simulink model "gm_sampleModel1849_sub"  (R2023a)
settings: Solver=VariableStepAuto  StartTime=0.0  StopTime=10.0  RelTol=1e-3
libraries: simulink x2
settings Model: Creator=user1  LastModifiedBy=user1
settings OptimizationCC: BlockReduction=off  ConditionallyExecuteInputs=off
settings DebuggingCC: InheritedTsInSrcMsg=none

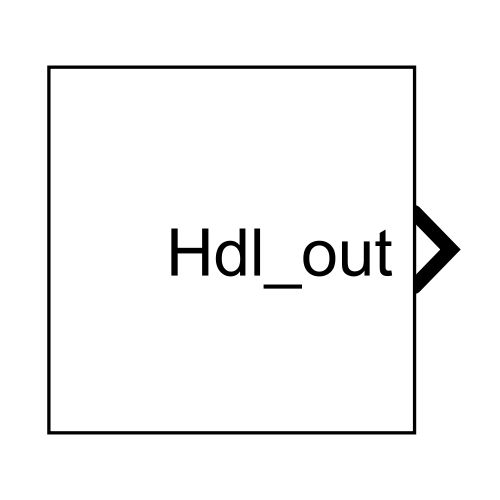
[thumbnail: Simulink's stored preview of the top-level diagram]
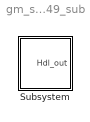
== system gm_sampleModel1849_sub ==
  Subsystem : Subsystem

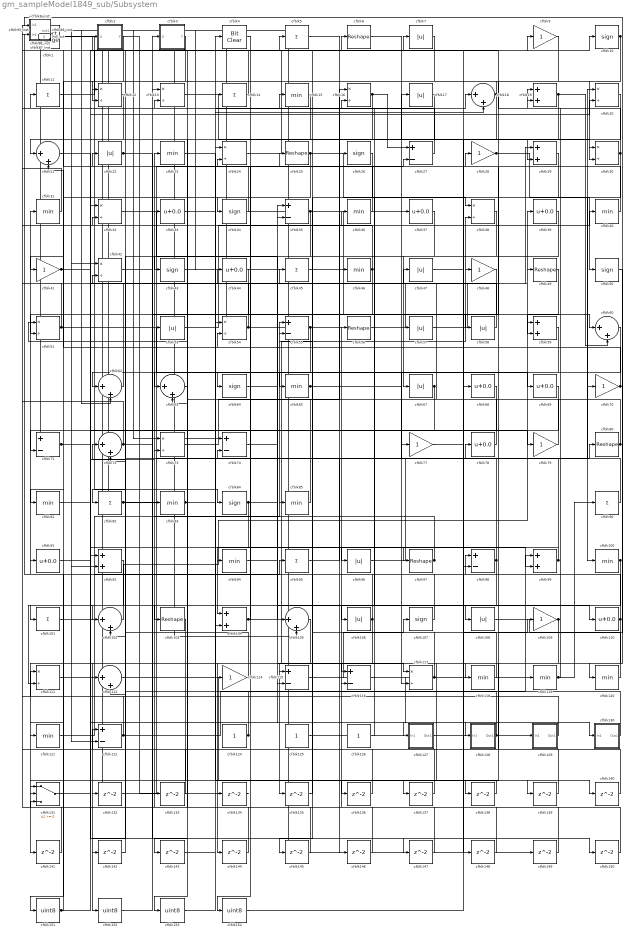
== system gm_sampleModel1849_sub/Subsystem ==
  cfblk1 : simulink/Logic and Bit Operations/Detect Change  vinit=0  OutDataTypeStr=uint8
      settings: LibrarySourceBlock=|
      | hdlsllib/Logic and Bit
      | Operations/Detect
      | Change
  cfblk{10,26,34,43,50,64,84,107} (8 alike) : Signum
  cfblk{15,23,31,36,40,46,65,81,83,85,94,100,118..121} (16 alike) : MinMax  OutDataTypeStr=uint8
  cfblk{5,11,14,45,82,90,95,101} (8 alike) : Sum  Inputs=+  OutDataTypeStr=uint8
  cfblk{18,21,60,62..63,72,102,105,112} (9 alike) : Sum  Inputs=|++  OutDataTypeStr=uint8
  cfblk{6,25,49,56,80,97,103} (7 alike) : Reshape
  cfblk{19,29,59,92,99,104} (6 alike) : Sum  OutDataTypeStr=uint8
  cfblk{7,17,22,47,53,57..58,67,96,106,108} (11 alike) : Abs  OutDataTypeStr=uint8  SaturateOnIntegerOverflow=off
  cfblk{9,28,41,48,70,77,79,109,114} (9 alike) : Gain  OutDataTypeStr=uint8
  cfblk{33,37,39,44,68..69,78,91,110} (9 alike) : Bias  Bias=0.0  SaturateOnIntegerOverflow=off
  cfblk{12..13,16,20,24,30,32,38,42,51,54,73,111,117} (14 alike) : Product  Inputs=*/  OutDataTypeStr=uint8  RndMeth=Zero  SaturateOnIntegerOverflow=on
  cfblk113_inst : Subsystem
  cfblk{27,35,55,71,74,98,115..116,122} (9 alike) : Sum  Inputs=+-  OutDataTypeStr=uint8
  cfblk124 : Constant  OutDataTypeStr=uint8  SampleTime=-1
  cfblk125 : Constant  OutDataTypeStr=uint8  SampleTime=-1
  cfblk126 : Constant  OutDataTypeStr=uint8  SampleTime=-1
  cfblk127 : Subsystem
  cfblk128 : Subsystem
  cfblk129 : Subsystem
  cfblk130 : Subsystem
  cfblk131 : Switch  OutDataTypeStr=uint8  SaturateOnIntegerOverflow=off  InputSameDT=off
  cfblk{132..150} (19 alike) : Delay  SampleTime=1
  cfblk{151..154} (4 alike) : DataTypeConversion  OutDataTypeStr=uint8  SaturateOnIntegerOverflow=off  RndMeth=Floor
  cfblk2 : Subsystem  mask(Detect Fall Nonpositive){vinit=double(0), InputProcessing=Elements as channels (sample based), OutDataTypeStr=uint8}
      mask prompts: vinit "Simulink:masks:InitialCondition_MP"; InputProcessing "Simulink:masks:InputProcessing_MP"; OutDataTypeStr "Simulink:masks:OutputDataType_MP"
      mask help: Simulink:masks:DetectFallNonpositive_MD
      mask init:
      | InputProcessing = 'Elements as channels (sample based)';
      | OutDataTypeStr = 'uint8';
      | vinit = double(0);
      mask TypeOptions InputProcessing: Simulink:masks:ColumnsAsChannelsFrameBased | Simulink:masks:ElementsAsChannelsSampleBased
      mask TypeOptions OutDataTypeStr: Simulink:masks:uint8 | Simulink:masks:boolean
      mask Display: fprintf('U <= 0\n&  NOT\nU/z <= 0')
  cfblk3 : Subsystem  mask(Detect Rise Positive){vinit=double(0), InputProcessing=Elements as channels (sample based), OutDataTypeStr=uint8}
      mask prompts: vinit "Simulink:masks:InitialCondition_MP"; InputProcessing "Simulink:masks:InputProcessing_MP"; OutDataTypeStr "Simulink:masks:OutputDataType_MP"
      mask help: Simulink:masks:DetectRisePositive_MD
      mask init:
      | InputProcessing = 'Elements as channels (sample based)';
      | OutDataTypeStr = 'uint8';
      | vinit = double(0);
      mask TypeOptions InputProcessing: Simulink:masks:ColumnsAsChannelsFrameBased | Simulink:masks:ElementsAsChannelsSampleBased
      mask TypeOptions OutDataTypeStr: Simulink:masks:uint8 | Simulink:masks:boolean
      mask Display: fprintf('U > 0\n&  NOT\nU/z > 0')
  cfblk4 : simulink/Logic and Bit Operations/Bit Clear  iBit=0
      settings: LibrarySourceBlock=|
      | hdlsllib/Logic and Bit
      | Operations/Bit Clear
  cfblk52_inst : Subsystem
  cfblk61_inst : Subsystem
  cfblk66_inst : Subsystem
  cfblk75_inst : Subsystem
  cfblk76_inst : Subsystem
  cfblk86_inst : Subsystem
  cfblk87_inst : Subsystem
  cfblk88_inst : Subsystem
  cfblk89_inst : Subsystem
  cfblk8_inst : Subsystem
  cfblk93_inst : Subsystem
  Hdl_out : Outport  OutDataTypeStr=uint8  SampleTime=1
  wires:
  cfblk1/1 -> cfblk84/1
  cfblk10/1 -> cfblk30/2, cfblk12/2
  cfblk100/1 -> cfblk112/2, cfblk108/1
  cfblk101/1 -> cfblk55/1
  cfblk102/1 -> cfblk39/1
  cfblk103/1 -> cfblk152/1
  cfblk104/1 -> cfblk35/2, cfblk38/2, cfblk24/2, cfblk117/1
  cfblk105/1 -> cfblk144/1
  cfblk106/1 -> cfblk141/1, cfblk31/1
  cfblk107/1 -> cfblk89_inst/2(in2)
  cfblk108/1 -> cfblk89_inst/1(in1)
  cfblk109/1 -> cfblk19/1, cfblk118/1
  cfblk11/1 -> cfblk6/1
  cfblk110/1 -> cfblk138/1, cfblk137/1, cfblk135/1, cfblk23/1, cfblk45/1
  cfblk111/1 -> cfblk132/1
  cfblk112/1 -> cfblk139/1
  cfblk113_inst/1(out1) -> cfblk129/1(In1)
  cfblk114/1 -> cfblk11/1
  cfblk115/1 -> cfblk107/1
  cfblk116/1 -> cfblk128/1(In1)
  cfblk117/1 -> cfblk74/2, cfblk109/1
  cfblk118/1 -> cfblk85/1
  cfblk119/1 -> cfblk19/2, cfblk90/1
  cfblk12/1 -> cfblk51/2
  cfblk120/1 -> cfblk78/1
  cfblk121/1 -> cfblk95/1
  cfblk122/1 -> cfblk99/1, cfblk88_inst/2(in2), cfblk8_inst/1(in1)
  cfblk124/1 -> cfblk32/2, cfblk13/2
  cfblk125/1 -> cfblk56/1
  cfblk126/1 -> cfblk16/2
  cfblk127/1(Out1) -> cfblk10/1
  cfblk128/1(Out1) -> cfblk22/1, cfblk5/1
  cfblk129/1(Out1) -> cfblk111/1
  cfblk13/1 -> cfblk146/1
  cfblk130/1(Out1) -> cfblk28/1
  cfblk131/1 -> cfblk48/1
  cfblk132/1 -> cfblk27/2
  cfblk133/1 -> cfblk122/1
  cfblk134/1 -> cfblk1/1
  cfblk135/1 -> cfblk55/2
  cfblk136/1 -> cfblk75_inst/2(in2)
  cfblk137/1 -> cfblk72/1
  cfblk138/1 -> cfblk131/2
  cfblk139/1 -> cfblk98/1
  cfblk14/1 -> cfblk88_inst/1(in1)
  cfblk140/1 -> cfblk93_inst/1(in1)
  cfblk141/1 -> cfblk52_inst/1(in1)
  cfblk142/1 -> cfblk102/2
  cfblk143/1 -> cfblk18/2
  cfblk144/1 -> cfblk73/1
  cfblk145/1 -> cfblk66_inst/2(in2)
  cfblk146/1 -> cfblk42/2
  cfblk147/1 -> cfblk63/2
  cfblk148/1 -> cfblk87_inst/1(in1)
  cfblk149/1 -> cfblk131/3
  cfblk15/1 -> cfblk121/1
  cfblk150/1 -> cfblk116/2
  cfblk151/1 -> cfblk91/1, cfblk73/2
  cfblk152/1 -> cfblk3/1(U)
  cfblk153/1 -> cfblk4/1
  cfblk154/1 -> cfblk68/1
  cfblk16/1 -> cfblk43/1, cfblk27/1
  cfblk17/1 -> cfblk34/1
  cfblk18/1 -> cfblk98/2, cfblk12/1
  cfblk19/1 -> cfblk60/2, cfblk143/1
  cfblk2/1(Y) -> cfblk21/1
  cfblk20/1 -> cfblk64/1
  cfblk21/1 -> cfblk96/1
  cfblk22/1 -> cfblk60/1, cfblk150/1
  cfblk23/1 -> cfblk136/1
  cfblk24/1 -> cfblk7/1
  cfblk25/1 -> cfblk41/1, cfblk38/1
  cfblk26/1 -> cfblk65/1
  cfblk27/1 -> cfblk75_inst/1(in1)
  cfblk28/1 -> cfblk50/1, cfblk70/1
  cfblk29/1 -> cfblk106/1
  cfblk3/1(Y) -> cfblk151/1
  cfblk30/1 -> cfblk52_inst/2(in2), cfblk145/1
  cfblk31/1 -> cfblk61_inst/1(in1)
  cfblk32/1 -> cfblk105/1
  cfblk33/1 -> cfblk18/1
  cfblk34/1 -> cfblk86_inst/1(in1)
  cfblk35/1 -> cfblk63/1, cfblk59/2
  cfblk36/1 -> cfblk24/1
  cfblk37/1 -> cfblk153/1
  cfblk38/1 -> cfblk112/1
  cfblk39/1 -> cfblk67/1
  cfblk4/1 -> cfblk154/1
  cfblk40/1 -> cfblk16/1
  cfblk41/1 -> cfblk92/1, cfblk127/1(In1)
  cfblk42/1 -> cfblk33/1
  cfblk43/1 -> cfblk14/1
  cfblk44/1 -> cfblk131/1
  cfblk45/1 -> cfblk100/1
  cfblk46/1 -> cfblk86_inst/2(in2), cfblk82/1
  cfblk47/1 -> cfblk140/1
  cfblk48/1 -> cfblk101/1
  cfblk49/1 -> cfblk59/1
  cfblk5/1 -> cfblk29/2
  cfblk50/1 -> cfblk120/1
  cfblk51/1 -> cfblk113_inst/2(in2), cfblk77/1
  cfblk52_inst/1(out1) -> cfblk93_inst/2(in2), cfblk53/1
  cfblk53/1 -> cfblk36/1
  cfblk54/1 -> cfblk8_inst/2(in2), cfblk116/1
  cfblk55/1 -> cfblk72/2, cfblk62/1
  cfblk56/1 -> cfblk49/1
  cfblk57/1 -> cfblk29/1
  cfblk58/1 -> cfblk32/1
  cfblk59/1 -> cfblk134/1
  cfblk6/1 -> cfblk30/1
  cfblk60/1 -> cfblk142/1
  cfblk61_inst/1(out1) -> cfblk133/1
  cfblk62/1 -> cfblk113_inst/1(in1)
  cfblk63/1 -> cfblk103/1
  cfblk64/1 -> cfblk110/1
  cfblk65/1 -> cfblk69/1, cfblk117/2
  cfblk66_inst/1(out1) -> cfblk87_inst/2(in2), cfblk37/1
  cfblk67/1 -> cfblk71/2, cfblk114/1
  cfblk68/1 -> cfblk115/1
  cfblk69/1 -> cfblk102/1
  cfblk7/1 -> cfblk81/1
  cfblk70/1 -> cfblk21/2, cfblk54/2
  cfblk71/1 -> cfblk79/1, cfblk147/1
  cfblk72/1 -> cfblk99/2, cfblk66_inst/1(in1)
  cfblk73/1 -> cfblk26/1
  cfblk74/1 -> cfblk115/2
  cfblk75_inst/1(out1) -> cfblk42/1
  cfblk76_inst/1(out1) -> cfblk57/1
  cfblk77/1 -> cfblk148/1
  cfblk78/1 -> cfblk2/1(U)
  cfblk79/1 -> cfblk13/1
  cfblk8_inst/1(out1) -> cfblk76_inst/1(in1), cfblk62/2, cfblk105/2
  cfblk80/1 -> cfblk76_inst/2(in2), cfblk47/1
  cfblk81/1 -> cfblk9/1
  cfblk82/1 -> cfblk17/1, cfblk54/1
  cfblk83/1 -> cfblk25/1, Hdl_out/1
  cfblk84/1 -> cfblk104/1, cfblk130/1(In1), cfblk40/1
  cfblk85/1 -> cfblk51/1
  cfblk86_inst/1(out1) -> cfblk71/1, cfblk149/1
  cfblk87_inst/1(out1) -> cfblk122/2, cfblk46/1
  cfblk88_inst/1(out1) -> cfblk74/1
  cfblk89_inst/1(out1) -> cfblk92/2
  cfblk9/1 -> cfblk58/1
  cfblk90/1 -> cfblk15/1
  cfblk91/1 -> cfblk20/2
  cfblk92/1 -> cfblk111/2
  cfblk93_inst/1(out1) -> cfblk119/1
  cfblk94/1 -> cfblk35/1
  cfblk95/1 -> cfblk80/1
  cfblk96/1 -> cfblk20/1
  cfblk97/1 -> cfblk83/1, cfblk94/1
  cfblk98/1 -> cfblk44/1, cfblk104/2
  cfblk99/1 -> cfblk97/1, cfblk61_inst/2(in2)

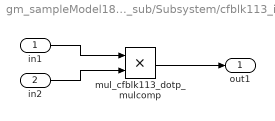
== system gm_sampleModel1849_sub/Subsystem/cfblk113_inst ==
  in1 : Inport  OutDataTypeStr=uint8  SampleTime=1
  in2 : Inport  Port=2  OutDataTypeStr=uint8  SampleTime=1
  mul_cfblk113_dotp_mulcomp : Product  Inputs=**  OutDataTypeStr=uint8  SampleTime=1
  out1 : Outport  OutDataTypeStr=uint8  SampleTime=1
  wires:
  in1/1 -> mul_cfblk113_dotp_mulcomp/1
  in2/1 -> mul_cfblk113_dotp_mulcomp/2
  mul_cfblk113_dotp_mulcomp/1 -> out1/1

== system gm_sampleModel1849_sub/Subsystem/cfblk127 ==
  In1 : Inport  OutDataTypeStr=uint8  PortDimensions=1  SampleTime=1
  Out1 : Outport  SampleTime=1
  wires:
  In1/1 -> Out1/1

== system gm_sampleModel1849_sub/Subsystem/cfblk128 ==
  In1 : Inport  OutDataTypeStr=uint8  PortDimensions=1  SampleTime=1
  Out1 : Outport  SampleTime=1
  wires:
  In1/1 -> Out1/1

== system gm_sampleModel1849_sub/Subsystem/cfblk129 ==
  In1 : Inport  OutDataTypeStr=uint8  PortDimensions=1  SampleTime=1
  Out1 : Outport  SampleTime=1
  wires:
  In1/1 -> Out1/1

== system gm_sampleModel1849_sub/Subsystem/cfblk130 ==
  In1 : Inport  OutDataTypeStr=uint8  PortDimensions=1  SampleTime=1
  Out1 : Outport  SampleTime=1
  wires:
  In1/1 -> Out1/1

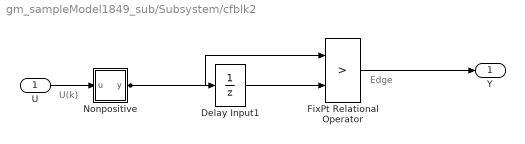
== system gm_sampleModel1849_sub/Subsystem/cfblk2 ==
  note: U(k)
  note: Edge
  U : Inport  OutDataTypeStr=uint8  SampleTime=1
  Delay Input1 : UnitDelay  Description=Store in Global RAM  DisableCoverage=on  InitialCondition=vinit  SampleTime=-1  HasFrameUpgradeWarning=on
  FixPt Relational Operator : RelationalOperator  Operator=>  OutDataTypeStr=fixdt(0, 8)  ZeroCross=off  InputSameDT=off
  Nonpositive : Subsystem  mask(Compare To Zero){relop=<=, OutDataTypeStr=boolean, ZeroCross=off}
      mask prompts: relop "Simulink:masks:Operator_MP"; OutDataTypeStr "Simulink:masks:OutputDataType_MP"; ZeroCross "Simulink:masks:EnableZerocrossingDetection_MP"
      mask help: Simulink:masks:CompareToZero_MD
      mask init:
      | OutDataTypeStr = 'boolean';
      | ZeroCross = 'off';
      | blkName = 'sampleModel1849_sub/Subsystem/cfblk2/Nonpositive';
      | relop = '<=';
      | setValue = 'boolean';
      mask TypeOptions relop: == | ~= | < | <= | >= | >
      mask TypeOptions OutDataTypeStr: Simulink:masks:uint8 | Simulink:masks:boolean
      mask Callback ZeroCross: sl('zeroCrossEnable', gcbh);
      mask Display: disp([relop,' 0'])
  Y : Outport  SampleTime=1
  wires:
  U/1 -> Nonpositive/1(u)
  Delay Input1/1 -> FixPt Relational Operator/2
  FixPt Relational Operator/1 -> Y/1
  Nonpositive/1(y) -> FixPt Relational Operator/1, Delay Input1/1

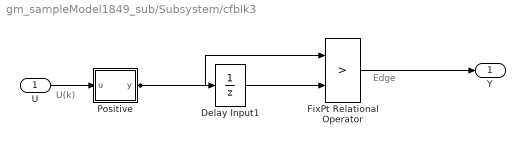
== system gm_sampleModel1849_sub/Subsystem/cfblk3 ==
  note: U(k)
  note: Edge
  U : Inport  OutDataTypeStr=uint8  SampleTime=1
  Delay Input1 : UnitDelay  Description=Store in Global RAM  DisableCoverage=on  InitialCondition=vinit  SampleTime=-1  HasFrameUpgradeWarning=on
  FixPt Relational Operator : RelationalOperator  Operator=>  OutDataTypeStr=fixdt(0, 8)  ZeroCross=off  InputSameDT=off
  Positive : Subsystem  mask(Compare To Zero){relop=>, OutDataTypeStr=boolean, ZeroCross=off}
      mask prompts: relop "Simulink:masks:Operator_MP"; OutDataTypeStr "Simulink:masks:OutputDataType_MP"; ZeroCross "Simulink:masks:EnableZerocrossingDetection_MP"
      mask help: Simulink:masks:CompareToZero_MD
      mask init:
      | OutDataTypeStr = 'boolean';
      | ZeroCross = 'off';
      | blkName = 'sampleModel1849_sub/Subsystem/cfblk3/Positive';
      | relop = '>';
      | setValue = 'boolean';
      mask TypeOptions relop: == | ~= | < | <= | >= | >
      mask TypeOptions OutDataTypeStr: Simulink:masks:uint8 | Simulink:masks:boolean
      mask Callback ZeroCross: sl('zeroCrossEnable', gcbh);
      mask Display: disp([relop,' 0'])
  Y : Outport  SampleTime=1
  wires:
  U/1 -> Positive/1(u)
  Delay Input1/1 -> FixPt Relational Operator/2
  FixPt Relational Operator/1 -> Y/1
  Positive/1(y) -> FixPt Relational Operator/1, Delay Input1/1

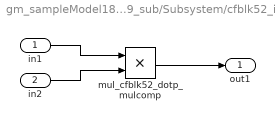
== system gm_sampleModel1849_sub/Subsystem/cfblk52_inst ==
  in1 : Inport  OutDataTypeStr=uint8  SampleTime=1
  in2 : Inport  Port=2  OutDataTypeStr=uint8  SampleTime=1
  mul_cfblk52_dotp_mulcomp : Product  Inputs=**  OutDataTypeStr=uint8  SampleTime=1
  out1 : Outport  OutDataTypeStr=uint8  SampleTime=1
  wires:
  in1/1 -> mul_cfblk52_dotp_mulcomp/1
  in2/1 -> mul_cfblk52_dotp_mulcomp/2
  mul_cfblk52_dotp_mulcomp/1 -> out1/1

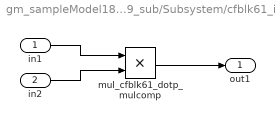
== system gm_sampleModel1849_sub/Subsystem/cfblk61_inst ==
  in1 : Inport  OutDataTypeStr=uint8  SampleTime=1
  in2 : Inport  Port=2  OutDataTypeStr=uint8  SampleTime=1
  mul_cfblk61_dotp_mulcomp : Product  Inputs=**  OutDataTypeStr=uint8  SampleTime=1
  out1 : Outport  OutDataTypeStr=uint8  SampleTime=1
  wires:
  in1/1 -> mul_cfblk61_dotp_mulcomp/1
  in2/1 -> mul_cfblk61_dotp_mulcomp/2
  mul_cfblk61_dotp_mulcomp/1 -> out1/1

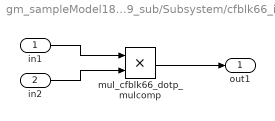
== system gm_sampleModel1849_sub/Subsystem/cfblk66_inst ==
  in1 : Inport  OutDataTypeStr=uint8  SampleTime=1
  in2 : Inport  Port=2  OutDataTypeStr=uint8  SampleTime=1
  mul_cfblk66_dotp_mulcomp : Product  Inputs=**  OutDataTypeStr=uint8  SampleTime=1
  out1 : Outport  OutDataTypeStr=uint8  SampleTime=1
  wires:
  in1/1 -> mul_cfblk66_dotp_mulcomp/1
  in2/1 -> mul_cfblk66_dotp_mulcomp/2
  mul_cfblk66_dotp_mulcomp/1 -> out1/1

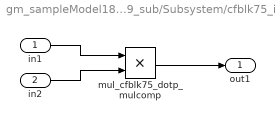
== system gm_sampleModel1849_sub/Subsystem/cfblk75_inst ==
  in1 : Inport  OutDataTypeStr=uint8  SampleTime=1
  in2 : Inport  Port=2  OutDataTypeStr=uint8  SampleTime=1
  mul_cfblk75_dotp_mulcomp : Product  Inputs=**  OutDataTypeStr=uint8  SampleTime=1
  out1 : Outport  OutDataTypeStr=uint8  SampleTime=1
  wires:
  in1/1 -> mul_cfblk75_dotp_mulcomp/1
  in2/1 -> mul_cfblk75_dotp_mulcomp/2
  mul_cfblk75_dotp_mulcomp/1 -> out1/1

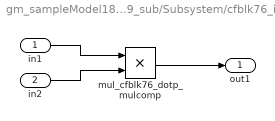
== system gm_sampleModel1849_sub/Subsystem/cfblk76_inst ==
  in1 : Inport  OutDataTypeStr=uint8  SampleTime=1
  in2 : Inport  Port=2  OutDataTypeStr=uint8  SampleTime=1
  mul_cfblk76_dotp_mulcomp : Product  Inputs=**  OutDataTypeStr=uint8  SampleTime=1
  out1 : Outport  OutDataTypeStr=uint8  SampleTime=1
  wires:
  in1/1 -> mul_cfblk76_dotp_mulcomp/1
  in2/1 -> mul_cfblk76_dotp_mulcomp/2
  mul_cfblk76_dotp_mulcomp/1 -> out1/1

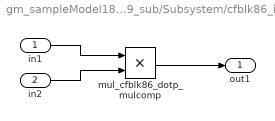
== system gm_sampleModel1849_sub/Subsystem/cfblk86_inst ==
  in1 : Inport  OutDataTypeStr=uint8  SampleTime=1
  in2 : Inport  Port=2  OutDataTypeStr=uint8  SampleTime=1
  mul_cfblk86_dotp_mulcomp : Product  Inputs=**  OutDataTypeStr=uint8  SampleTime=1
  out1 : Outport  OutDataTypeStr=uint8  SampleTime=1
  wires:
  in1/1 -> mul_cfblk86_dotp_mulcomp/1
  in2/1 -> mul_cfblk86_dotp_mulcomp/2
  mul_cfblk86_dotp_mulcomp/1 -> out1/1

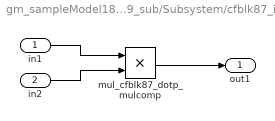
== system gm_sampleModel1849_sub/Subsystem/cfblk87_inst ==
  in1 : Inport  OutDataTypeStr=uint8  SampleTime=1
  in2 : Inport  Port=2  OutDataTypeStr=uint8  SampleTime=1
  mul_cfblk87_dotp_mulcomp : Product  Inputs=**  OutDataTypeStr=uint8  SampleTime=1
  out1 : Outport  OutDataTypeStr=uint8  SampleTime=1
  wires:
  in1/1 -> mul_cfblk87_dotp_mulcomp/1
  in2/1 -> mul_cfblk87_dotp_mulcomp/2
  mul_cfblk87_dotp_mulcomp/1 -> out1/1

== system gm_sampleModel1849_sub/Subsystem/cfblk88_inst ==
  in1 : Inport  OutDataTypeStr=uint8  SampleTime=1
  in2 : Inport  Port=2  OutDataTypeStr=uint8  SampleTime=1
  mul_cfblk88_dotp_mulcomp : Product  Inputs=**  OutDataTypeStr=uint8  SampleTime=1
  out1 : Outport  OutDataTypeStr=uint8  SampleTime=1
  wires:
  in1/1 -> mul_cfblk88_dotp_mulcomp/1
  in2/1 -> mul_cfblk88_dotp_mulcomp/2
  mul_cfblk88_dotp_mulcomp/1 -> out1/1

== system gm_sampleModel1849_sub/Subsystem/cfblk89_inst ==
  in1 : Inport  OutDataTypeStr=uint8  SampleTime=1
  in2 : Inport  Port=2  OutDataTypeStr=uint8  SampleTime=1
  mul_cfblk89_dotp_mulcomp : Product  Inputs=**  OutDataTypeStr=uint8  SampleTime=1
  out1 : Outport  OutDataTypeStr=uint8  SampleTime=1
  wires:
  in1/1 -> mul_cfblk89_dotp_mulcomp/1
  in2/1 -> mul_cfblk89_dotp_mulcomp/2
  mul_cfblk89_dotp_mulcomp/1 -> out1/1

== system gm_sampleModel1849_sub/Subsystem/cfblk8_inst ==
  in1 : Inport  OutDataTypeStr=uint8  SampleTime=1
  in2 : Inport  Port=2  OutDataTypeStr=uint8  SampleTime=1
  mul_cfblk8_dotp_mulcomp : Product  Inputs=**  OutDataTypeStr=uint8  SampleTime=1
  out1 : Outport  OutDataTypeStr=uint8  SampleTime=1
  wires:
  in1/1 -> mul_cfblk8_dotp_mulcomp/1
  in2/1 -> mul_cfblk8_dotp_mulcomp/2
  mul_cfblk8_dotp_mulcomp/1 -> out1/1

== system gm_sampleModel1849_sub/Subsystem/cfblk93_inst ==
  in1 : Inport  OutDataTypeStr=uint8  SampleTime=1
  in2 : Inport  Port=2  OutDataTypeStr=uint8  SampleTime=1
  mul_cfblk93_dotp_mulcomp : Product  Inputs=**  OutDataTypeStr=uint8  SampleTime=1
  out1 : Outport  OutDataTypeStr=uint8  SampleTime=1
  wires:
  in1/1 -> mul_cfblk93_dotp_mulcomp/1
  in2/1 -> mul_cfblk93_dotp_mulcomp/2
  mul_cfblk93_dotp_mulcomp/1 -> out1/1

== system gm_sampleModel1849_sub/Subsystem/cfblk2/Nonpositive ==
  u : Inport  OutDataTypeStr=uint8  SampleTime=1
  Compare : RelationalOperator  Operator=<=  OutDataTypeStr=boolean  ZeroCross=off
  Constant : Constant  DisableCoverage=on  Value=0  OutDataTypeStr=Inherit: Inherit via back propagation  SampleTime=-1  PreserveConstantTs=on
  y : Outport  SampleTime=1
  wires:
  u/1 -> Compare/1
  Compare/1 -> y/1
  Constant/1 -> Compare/2

== system gm_sampleModel1849_sub/Subsystem/cfblk3/Positive ==
  u : Inport  OutDataTypeStr=uint8  SampleTime=1
  Compare : RelationalOperator  Operator=>  OutDataTypeStr=boolean  ZeroCross=off
  Constant : Constant  DisableCoverage=on  Value=0  OutDataTypeStr=Inherit: Inherit via back propagation  SampleTime=-1  PreserveConstantTs=on
  y : Outport  SampleTime=1
  wires:
  u/1 -> Compare/1
  Compare/1 -> y/1
  Constant/1 -> Compare/2
